simulink model "test_loopback_buf"  (Simulink 6.2)
settings: Solver=ode45  StartTime=0.0  StopTime=4000  RelTol=1e-3
undefined symbols (not defined in the file): Down, Up
libraries: xbsIndex_r3 x1383, xps_library x52, casper_library x37
(part 1 of 8)
settings Model: LastModifiedBy=dsp
settings DebuggingCC: SolverPrmCheckMsg=warning

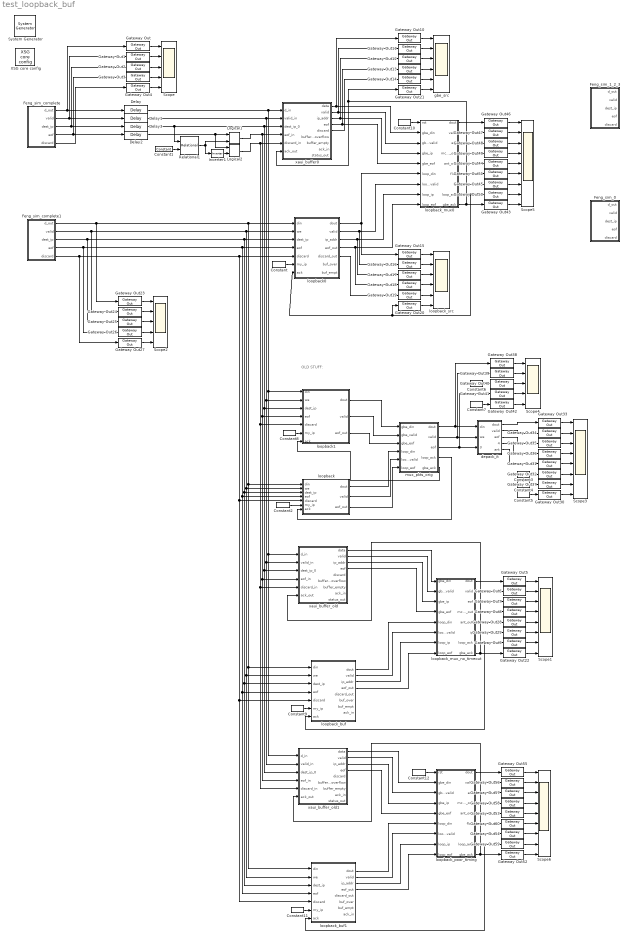
== system test_loopback_buf ==
  note: OLD STUFF:
  " System Generator" : xbsIndex_r3/ System Generator  Tag=genX  xilinxfamily=Virtex2P  part=xc2vp70  speed=-7  package=ff1704  synthesis_tool=XST  directory=./b_2x_8a_r308d/sysgen  testbench=off  simulink_period=1  sysclk_period=4.878  incr_netlist=off  trim_vbits=Everywhere in SubSystem  dbl_ovrd=According to Block Masks  core_generation=According to Block Masks  run_coregen=off  deprecated_control=off  eval_field=0
      settings: AttributesFormatString=System\nGenerator
  Constant{,1..12} (13 alike) : xbsIndex_r3/Constant  const=0  equ=P=C  arith_type=Unsigned  n_bits=1  bin_pt=0  opselect=C  inp2=PCIN>>17  opr=+  inp1=P  carry=CIN  iostate=0  explicit_period=on  period=1  dbl_ovrd=off
  Delay{,1..3} (4 alike) : xbsIndex_r3/Delay  latency=220  reg_retiming=off  explicit_period=off  period=1  en=off  accept_only_valid=off  init_zero=on  dbl_ovrd=off  show_param=off
      settings: xl_area=[0, 0, 0, 0, 0, 0, 0]
  Feng_sim_0 : Subsystem
  Feng_sim_1_2_3 : Subsystem
  Feng_sim_complete : Subsystem
  Feng_sim_complete1 : Subsystem
  Gateway Out{,1..60} (61 alike) : xbsIndex_r3/Gateway Out  output_type=Double  nbits=8  bin_pt=6  arith_type=Boolean  quantization=Truncate  overflow=Wrap  hdl_port=on  timing_constraint=None  locs_specified=off  LOCs={}  needs_fixed_name=off  show_param=off
      settings: xl_area=[0, 0, 0, 0, 0, 0, 0]
  Inverter1 : xbsIndex_r3/Inverter  latency=0  explicit_period=off  period=1  en=off  dbl_ovrd=off  show_param=off
      settings: xl_area=[0, 0, 0, 0, 0, 0, 0]
  Logical1 : xbsIndex_r3/Logical  logical_function=AND  inputs=2  precision=Full  arith_type=Unsigned  n_bits=8  bin_pt=2  align_bp=on  latency=0  explicit_period=off  period=1  en=off  dbl_ovrd=off  show_param=off
      settings: xl_area=[0, 0, 0, 0, 0, 0, 0]
  Logical2 : xbsIndex_r3/Logical  logical_function=AND  inputs=2  precision=Full  arith_type=Unsigned  n_bits=8  bin_pt=2  align_bp=on  latency=0  explicit_period=off  period=1  en=off  dbl_ovrd=off  show_param=off
      settings: xl_area=[0, 0, 0, 0, 0, 0, 0]
  Relational1 : xbsIndex_r3/Relational  mode=a!=b  latency=0  explicit_period=off  period=1  en=off  dbl_ovrd=off  show_param=off
      settings: xl_area=[0, 0, 0, 0, 0, 0, 0]
  Scope : Scope  NumInputPorts=5
      settings: TimeRange=10000  YMin=0~0~0~0~-1  YMax=5000~1~3~1~1
  Scope1 : Scope  NumInputPorts=8
      settings: YMin=1100~0~0~-1~0.95~-5~-5~-5  YMax=1200~1~1~1~1.05~5~5~5  SaveName=ScopeData19
  Scope2 : Scope  NumInputPorts=5
      settings: TimeRange=10000  YMin=0~0~0~0~-1  YMax=5000~1~3~1~1  SaveName=ScopeData12
  Scope3 : Scope  NumInputPorts=8
      settings: YMin=1100~0~0~-1~0.95~-5~-5~-5  YMax=1200~1~1~1~1.05~5~5~5  SaveName=ScopeData10
  Scope4 : Scope  NumInputPorts=5
      settings: TimeRange=10000  YMin=0~0~0~0~-1  YMax=5000~1~3~1~1  SaveName=ScopeData16
  Scope5 : Scope  NumInputPorts=9
      settings: YMin=1100~0~0~-1~0.95~-5~-5~-5~-5  YMax=1200~1~1~1~1.05~5~5~5~5  SaveName=ScopeData17
  Scope6 : Scope  NumInputPorts=9
      settings: YMin=1100~0~0~-1~0.95~-5~-5~-5~-5  YMax=1200~1~1~1~1.05~5~5~5~5  SaveName=ScopeData20
  XSG core config : xps_library/XSG core config  Tag=xps:xsg  hw_sys=BEE2_usr  ibob_linux=off  clk_src=sys_clk2x  gpio_clk_io_group=iBOB:sma  gpio_clk_bit_index=0  clk_rate=205  sample_period=1  synthesis_tool=XST  mpc_type=powerpc405
  depack_it : Subsystem  mask{payload_len=50}
      mask prompts: payload_len "Payload Length"
      mask init:
      | payload_bits = ceil(log2(payload_len));
      | packet_len = payload_len + 1;
      | packet_bits = ceil(log2(packet_len));
  gbe_src : Scope  NumInputPorts=6
      settings: YMin=95.95~0.95~1.9~-1~-1~-1  YMax=106.05~1.05~2.1~1~1~1  SaveName=ScopeData4
  loopback : Subsystem  mask{depth_bits=8}
      mask prompts: depth_bits "Buffer Size (2^?):"
      mask help: A loopback is a buffer for holding packets which are to be transmitted to one's self. Most switches drop any packets which have a destination IP address equal to the address of the transmitter. Thus, a seperate buffer is needed to collect these packets for readback.
  loopback0 : Subsystem  mask{depth_bits=10}
      mask prompts: depth_bits "Buffer Size (2^?):"
      mask help: A loopback is a buffer for holding packets which are to be transmitted to one's self. Most switches drop any packets which have a destination IP address equal to the address of the transmitter. Thus, a seperate buffer is needed to collect these packets for readback.
  loopback1 : Subsystem  mask{depth_bits=8}
      mask prompts: depth_bits "Buffer Size (2^?):"
      mask help: A loopback is a buffer for holding packets which are to be transmitted to one's self. Most switches drop any packets which have a destination IP address equal to the address of the transmitter. Thus, a seperate buffer is needed to collect these packets for readback.
  loopback_buf : Subsystem  mask{depth_bits=10}
      mask prompts: depth_bits "Buffer Size (2^?):"
      mask help: A loopback is a buffer for holding packets which are to be transmitted to one's self. Most switches drop any packets which have a destination IP address equal to the address of the transmitter. Thus, a seperate buffer is needed to collect these packets for readback.
  loopback_buf1 : Subsystem  mask{depth_bits=10}
      mask prompts: depth_bits "Buffer Size (2^?):"
      mask help: A loopback is a buffer for holding packets which are to be transmitted to one's self. Most switches drop any packets which have a destination IP address equal to the address of the transmitter. Thus, a seperate buffer is needed to collect these packets for readback.
  loopback_mux0 : Subsystem  mask{timeout_bits=27, payload_len=32}
      mask prompts: timeout_bits "Timeout (clock cycles, 2^?)"; payload_len "Expected payload length (in 64bit words)"
      mask init:
      | fmtstr = sprintf('Payload Len: %i', payload_len);
      | set_param(gcb, 'AttributesFormatString', fmtstr);
      settings: AttributesFormatString=Payload Len: 32
  loopback_mux_no_timeout : Subsystem  mask{loopback_timeout=20}
      mask prompts: loopback_timeout "loopback timeout (2^? clocks)"
  loopback_poor_timing : Subsystem  mask{timeout_bits=27, payload_len=50}
      mask prompts: timeout_bits "Timeout (clock cycles, 2^?)"; payload_len "Expected payload length (in 64bit words)"
      mask init:
      | fmtstr = sprintf('Payload Len: %i', payload_len);
      | set_param(gcb, 'AttributesFormatString', fmtstr);
      settings: AttributesFormatString=Payload Len: 50
  loopback_src : Scope  NumInputPorts=6
      settings: YMin=1500~0~1.59383e+008~0~-1~-5  YMax=3000~1~1.76161e+008~1~1~5  SaveName=ScopeData5
  mux_pkts_orig : Subsystem
  xaui_buffer0 : Subsystem  mask(mux_packets){depth_data_bits=10, depth_hdr_bits=5}
      mask prompts: depth_data_bits "Depth contents (2^?)"; depth_hdr_bits "Maximum number of packets to buffer? (2^?)"
      mask help: This block allows you to buffer a 10GbE datastream.
      mask init:
      | fmtstr = sprintf('Max %d data words.\nMax %d pkts.', 2^depth_data_bits,2^depth_hdr_bits);
      | set_param(gcb, 'AttributesFormatString', fmtstr);
      settings: AttributesFormatString=|
      | Max 1024 data words.
      | Max 32 pkts.
  xaui_buffer_old : Subsystem  mask(mux_packets){depth_data_bits=10, depth_hdr_bits=8}
      mask prompts: depth_data_bits "Depth contents (2^?)"; depth_hdr_bits "Maximum number of packets to buffer? (2^?)"
      mask help: This block allows you to buffer a 10GbE datastream.
      mask init:
      | fmtstr = sprintf('Max %d data words.\nMax %d pkts.', 2^depth_data_bits,2^depth_hdr_bits);
      | set_param(gcb, 'AttributesFormatString', fmtstr);
      settings: AttributesFormatString=|
      | Max 1024 data words.
      | Max 256 pkts.
  xaui_buffer_old1 : Subsystem  mask(mux_packets){depth_data_bits=10, depth_hdr_bits=8}
      mask prompts: depth_data_bits "Depth contents (2^?)"; depth_hdr_bits "Maximum number of packets to buffer? (2^?)"
      mask help: This block allows you to buffer a 10GbE datastream.
      mask init:
      | fmtstr = sprintf('Max %d data words.\nMax %d pkts.', 2^depth_data_bits,2^depth_hdr_bits);
      | set_param(gcb, 'AttributesFormatString', fmtstr);
      settings: AttributesFormatString=|
      | Max 1024 data words.
      | Max 256 pkts.
  wires:
  Feng_sim_complete/1(d_out) -> Gateway Out/1, Delay/1
  Feng_sim_complete/2(valid) -> Gateway Out1/1, Delay1/1
  Feng_sim_complete/4(eof) -> Gateway Out3/1, Delay2/1
  Feng_sim_complete/3(dest_ip) -> Gateway Out2/1, Delay3/1
  Feng_sim_complete/5(discard) -> Gateway Out4/1
  Gateway Out/1 -> Scope/1
  Gateway Out1/1 -> Scope/2
  Gateway Out2/1 -> Scope/3
  Gateway Out3/1 -> Scope/4
  Gateway Out4/1 -> Scope/5
  Delay/1 -> loopback1/1(din), xaui_buffer_old/1(d_in), xaui_buffer_old1/1(d_in), xaui_buffer0/1(d_in)
  Delay1/1 -> loopback1/2(we), xaui_buffer_old/2(valid_in), xaui_buffer_old1/2(valid_in), xaui_buffer0/2(valid_in)
  Delay3/1 -> Relational1/1, loopback1/3(dest_ip), xaui_buffer_old/3(dest_ip_0), xaui_buffer_old1/3(dest_ip_0), xaui_buffer0/3(dest_ip_0)
  Inverter1/1 -> Logical2/2
  Relational1/1 -> Inverter1/1, Logical1/2
  Logical1/1 -> loopback1/4(eof), xaui_buffer_old/4(eof_in), xaui_buffer_old1/4(eof_in), xaui_buffer0/4(eof_in)
  Logical2/1 -> loopback1/5(discard), xaui_buffer_old/5(discard_in), xaui_buffer_old1/5(discard_in), xaui_buffer0/5(discard_in)
  Constant1/1 -> Relational1/2
  Delay2/1 -> Logical1/1, Logical2/1
  Gateway Out10/1 -> gbe_src/1
  Gateway Out11/1 -> gbe_src/2
  Gateway Out12/1 -> gbe_src/3
  Gateway Out13/1 -> gbe_src/4
  Gateway Out14/1 -> gbe_src/5
  Gateway Out21/1 -> gbe_src/6
  Constant/1 -> loopback0/6(my_ip)
  Feng_sim_complete1/1(d_out) -> Gateway Out23/1, loopback/1(din), loopback_buf/1(din), loopback_buf1/1(din), loopback0/1(din)
  Feng_sim_complete1/2(valid) -> Gateway Out24/1, loopback/2(we), loopback_buf/2(we), loopback_buf1/2(we), loopback0/2(we)
  Feng_sim_complete1/3(dest_ip) -> Gateway Out25/1, loopback/3(dest_ip), loopback_buf/3(dest_ip), loopback_buf1/3(dest_ip), loopback0/3(dest_ip)
  Feng_sim_complete1/4(eof) -> Gateway Out26/1, loopback/4(eof), loopback_buf/4(eof), loopback_buf1/4(eof), loopback0/4(eof)
  Feng_sim_complete1/5(discard) -> Gateway Out27/1, loopback/5(discard), loopback_buf/5(discard), loopback_buf1/5(discard), loopback0/5(discard)
  Gateway Out23/1 -> Scope2/1
  Gateway Out24/1 -> Scope2/2
  Gateway Out25/1 -> Scope2/3
  Gateway Out26/1 -> Scope2/4
  Gateway Out27/1 -> Scope2/5
  mux_pkts_orig/1(dout) -> depack_it/1(din), Gateway Out38/1
  mux_pkts_orig/2(valid) -> depack_it/2(we), Gateway Out39/1
  mux_pkts_orig/3(eof) -> depack_it/3(eof_in), Gateway Out41/1
  loopback/1(dout) -> mux_pkts_orig/4(loop_din)
  loopback/2(valid) -> mux_pkts_orig/5(loop_valid)
  loopback/3(eof_out) -> mux_pkts_orig/6(loop_eof)
  mux_pkts_orig/4(loop_ack) -> loopback/7(ack)
  loopback1/1(dout) -> mux_pkts_orig/1(gbe_din)
  loopback1/2(valid) -> mux_pkts_orig/2(gbe_valid)
  loopback1/3(eof_out) -> mux_pkts_orig/3(gbe_eof)
  Constant2/1 -> loopback/6(my_ip)
  Gateway Out33/1 -> Scope3/1
  Gateway Out34/1 -> Scope3/2
  Gateway Out35/1 -> Scope3/3
  Gateway Out36/1 -> Scope3/4
  Gateway Out31/1 -> Scope3/5
  Gateway Out32/1 -> Scope3/6
  Gateway Out37/1 -> Scope3/7
  Gateway Out30/1 -> Scope3/8
  depack_it/1(dout) -> Gateway Out33/1
  depack_it/2(valid) -> Gateway Out34/1
  depack_it/3(eof) -> Gateway Out35/1
  depack_it/4(mcnt) -> Gateway Out36/1
  depack_it/5(ant) -> Gateway Out31/1
  Constant3/1 -> Gateway Out32/1
  Constant4/1 -> Gateway Out37/1
  Constant5/1 -> Gateway Out30/1
  Gateway Out38/1 -> Scope4/1
  Gateway Out39/1 -> Scope4/2
  Gateway Out40/1 -> Scope4/3
  Gateway Out41/1 -> Scope4/4
  Gateway Out42/1 -> Scope4/5
  Constant6/1 -> Gateway Out40/1
  Constant7/1 -> Gateway Out42/1
  Constant8/1 -> loopback1/6(my_ip)
  mux_pkts_orig/5(gbe_ack) -> loopback1/7(ack)
  Constant9/1 -> loopback_buf/6(my_ip)
  Gateway Out46/1 -> Scope5/1
  Gateway Out47/1 -> Scope5/2
  Gateway Out48/1 -> Scope5/3
  Gateway Out49/1 -> Scope5/4
  Gateway Out44/1 -> Scope5/5
  xaui_buffer0/1(data) -> Gateway Out10/1, loopback_mux0/2(gbe_din)
  xaui_buffer0/2(valid) -> Gateway Out11/1, loopback_mux0/3(gbe_valid)
  xaui_buffer0/3(ip_addr) -> Gateway Out12/1, loopback_mux0/4(gbe_ip)
  xaui_buffer0/4(eof) -> Gateway Out13/1, loopback_mux0/5(gbe_eof)
  loopback0/1(dout) -> Gateway Out15/1, loopback_mux0/6(loop_din)
  loopback0/2(valid) -> Gateway Out16/1, loopback_mux0/7(loop_valid)
  loopback0/3(ip_addr) -> Gateway Out17/1, loopback_mux0/8(loop_ip)
  loopback0/4(eof_out) -> Gateway Out18/1, loopback_mux0/9(loop_eof)
  Constant10/1 -> loopback_mux0/1(rst)
  Gateway Out5/1 -> Scope1/1
  Gateway Out6/1 -> Scope1/2
  Gateway Out7/1 -> Scope1/3
  xaui_buffer_old/1(data) -> loopback_mux_no_timeout/1(gbe_din)
  xaui_buffer_old/2(valid) -> loopback_mux_no_timeout/2(gbe_valid)
  xaui_buffer_old/4(eof) -> loopback_mux_no_timeout/4(gbe_eof)
  xaui_buffer_old/3(ip_addr) -> loopback_mux_no_timeout/3(gbe_ip)
  loopback_buf/2(valid) -> loopback_mux_no_timeout/6(loop_valid)
  loopback_buf/3(ip_addr) -> loopback_mux_no_timeout/7(loop_ip)
  loopback_buf/4(eof_out) -> loopback_mux_no_timeout/8(loop_eof)
  loopback_mux_no_timeout/7(loop_ack) -> Gateway Out9/1, loopback_buf/7(ack)
  loopback_mux_no_timeout/8(gbe_ack) -> Gateway Out22/1, xaui_buffer_old/6(ack_out)
  loopback_mux_no_timeout/1(dout) -> Gateway Out5/1
  loopback_mux_no_timeout/2(valid) -> Gateway Out6/1
  loopback_mux_no_timeout/3(eof) -> Gateway Out7/1
  Gateway Out8/1 -> Scope1/4
  Gateway Out28/1 -> Scope1/5
  Gateway Out29/1 -> Scope1/6
  Gateway Out9/1 -> Scope1/7
  Gateway Out22/1 -> Scope1/8
  loopback_mux_no_timeout/4(mcnt_out) -> Gateway Out8/1
  loopback_mux_no_timeout/5(ant_out) -> Gateway Out28/1
  loopback_mux_no_timeout/6(ip) -> Gateway Out29/1
  xaui_buffer0/5(discard) -> Gateway Out14/1
  loopback_buf/1(dout) -> loopback_mux_no_timeout/5(loop_din)
  Gateway Out15/1 -> loopback_src/1
  Gateway Out16/1 -> loopback_src/2
  Gateway Out17/1 -> loopback_src/3
  Gateway Out18/1 -> loopback_src/4
  Gateway Out19/1 -> loopback_src/5
  Gateway Out20/1 -> loopback_src/6
  Gateway Out51/1 -> Scope5/6
  Gateway Out45/1 -> Scope5/7
  Gateway Out50/1 -> Scope5/8
  Gateway Out43/1 -> Scope5/9
  loopback_mux0/1(dout) -> Gateway Out46/1
  loopback_mux0/2(valid) -> Gateway Out47/1
  loopback_mux0/3(eof) -> Gateway Out48/1
  loopback_mux0/4(mcnt_out) -> Gateway Out49/1
  loopback_mux0/5(ant_out) -> Gateway Out44/1
  loopback_mux0/6(flag) -> Gateway Out51/1
  loopback_mux0/7(ip) -> Gateway Out45/1
  loopback_mux0/8(loop_ack) -> Gateway Out50/1, Gateway Out20/1, loopback0/7(ack)
  loopback_mux0/9(gbe_ack) -> Gateway Out43/1, Gateway Out21/1, xaui_buffer0/6(ack_out)
  Constant11/1 -> loopback_buf1/6(my_ip)
  xaui_buffer_old1/1(data) -> loopback_poor_timing/2(gbe_din)
  xaui_buffer_old1/2(valid) -> loopback_poor_timing/3(gbe_valid)
  xaui_buffer_old1/4(eof) -> loopback_poor_timing/5(gbe_eof)
  xaui_buffer_old1/3(ip_addr) -> loopback_poor_timing/4(gbe_ip)
  loopback_poor_timing/8(loop_ack) -> loopback_buf1/7(ack), Gateway Out59/1
  loopback_poor_timing/9(gbe_ack) -> xaui_buffer_old1/6(ack_out), Gateway Out52/1
  loopback_buf1/2(valid) -> loopback_poor_timing/7(loop_valid)
  loopback_buf1/3(ip_addr) -> loopback_poor_timing/8(loop_ip)
  loopback_buf1/4(eof_out) -> loopback_poor_timing/9(loop_eof)
  loopback_buf1/1(dout) -> loopback_poor_timing/6(loop_din)
  Gateway Out55/1 -> Scope6/1
  Gateway Out56/1 -> Scope6/2
  Gateway Out57/1 -> Scope6/3
  Gateway Out58/1 -> Scope6/4
  Gateway Out53/1 -> Scope6/5
  Gateway Out60/1 -> Scope6/6
  Gateway Out54/1 -> Scope6/7
  Gateway Out59/1 -> Scope6/8
  Gateway Out52/1 -> Scope6/9
  Constant12/1 -> loopback_poor_timing/1(rst)
  loopback_poor_timing/1(dout) -> Gateway Out55/1
  loopback_poor_timing/2(valid) -> Gateway Out56/1
  loopback_poor_timing/3(eof) -> Gateway Out57/1
  loopback_poor_timing/4(mcnt_out) -> Gateway Out58/1
  loopback_poor_timing/5(ant_out) -> Gateway Out53/1
  loopback_poor_timing/6(flag) -> Gateway Out60/1
  loopback_poor_timing/7(ip) -> Gateway Out54/1
  loopback0/5(discard_out) -> Gateway Out19/1

== system test_loopback_buf/Feng_sim_0 ==
  Concat1 : xbsIndex_r3/Concat  num_inputs=3  explicit_period=off  period=1  dbl_ovrd=off
  Constant : xbsIndex_r3/Constant  const=0  equ=P=C  arith_type=Boolean  n_bits=1  bin_pt=0  opselect=C  inp2=PCIN>>17  opr=+  inp1=P  carry=CIN  iostate=0  explicit_period=on  period=1  dbl_ovrd=off
  Constant1 : xbsIndex_r3/Constant  const=1  equ=P=C  arith_type=Boolean  n_bits=1  bin_pt=0  opselect=C  inp2=PCIN>>17  opr=+  inp1=P  carry=CIN  iostate=0  explicit_period=off  period=1  dbl_ovrd=off
  Constant2 : Constant
  Constant3 : xbsIndex_r3/Constant  const=0  equ=P=C  arith_type=Boolean  n_bits=1  bin_pt=0  opselect=C  inp2=PCIN>>17  opr=+  inp1=P  carry=CIN  iostate=0  explicit_period=off  period=1  dbl_ovrd=off
  Constant4 : xbsIndex_r3/Constant  const=0  equ=P=C  arith_type=Unsigned  n_bits=32  bin_pt=0  opselect=C  inp2=PCIN>>17  opr=+  inp1=P  carry=CIN  iostate=0  explicit_period=on  period=1  dbl_ovrd=off
  Constant5 : xbsIndex_r3/Constant  const=0  equ=P=C  arith_type=Unsigned  n_bits=16-2  bin_pt=0  opselect=C  inp2=PCIN>>17  opr=+  inp1=P  carry=CIN  iostate=0  explicit_period=on  period=1  dbl_ovrd=off
  Constant6 : xbsIndex_r3/Constant  const=0  equ=P=C  arith_type=Unsigned  n_bits=32  bin_pt=0  opselect=C  inp2=PCIN>>17  opr=+  inp1=P  carry=CIN  iostate=0  explicit_period=on  period=1  dbl_ovrd=off
  Convert1 : xbsIndex_r3/Convert  arith_type=Boolean  n_bits=8  bin_pt=6  quantization=Truncate  overflow=Wrap  latency=0  explicit_period=on  period=1  dbl_ovrd=off  show_param=off  inserted_by_tool=off  pipeline=off
      settings: xl_area=[0, 0, 0, 0, 0, 0, 0]
  Convert2 : xbsIndex_r3/Convert  arith_type=Boolean  n_bits=8  bin_pt=6  quantization=Truncate  overflow=Wrap  latency=0  explicit_period=on  period=1  dbl_ovrd=off  show_param=off  inserted_by_tool=off  pipeline=off
      settings: xl_area=[0, 0, 0, 0, 0, 0, 0]
  Convert3 : xbsIndex_r3/Convert  arith_type=Boolean  n_bits=8  bin_pt=6  quantization=Truncate  overflow=Wrap  latency=0  explicit_period=on  period=1  dbl_ovrd=off  show_param=off  inserted_by_tool=off  pipeline=off
      settings: xl_area=[0, 0, 0, 0, 0, 0, 0]
  Counter1 : xbsIndex_r3/Counter  cnt_type=Free Running  n_bits=64  bin_pt=0  arith_type=Unsigned  start_count=0  cnt_to=Inf  cnt_by_val=1  operation=Up  explicit_period=off  period=1  load_pin=off  rst=on  en=on  dbl_ovrd=off  show_param=off  use_rpm=off  gen_core=off
      settings: xl_area=[0, 0, 0, 0, 0, 0, 0]
  Counter2 : xbsIndex_r3/Counter  cnt_type=Free Running  n_bits=32  bin_pt=0  arith_type=Unsigned  start_count=1  cnt_to=Inf  cnt_by_val=1  operation=Up  explicit_period=on  period=1  load_pin=off  rst=on  en=off  dbl_ovrd=off  show_param=off  use_rpm=on  gen_core=off
      settings: xl_area=[0, 0, 0, 0, 0, 0, 0]
  Counter3 : xbsIndex_r3/Counter  cnt_type=Free Running  n_bits=32  bin_pt=0  arith_type=Unsigned  start_count=0  cnt_to=1023  cnt_by_val=1  operation=Up  explicit_period=on  period=1  load_pin=off  rst=on  en=on  dbl_ovrd=off  show_param=off  use_rpm=on  gen_core=off
      settings: xl_area=[0, 0, 0, 0, 0, 0, 0]
  Delay{1..2,4..5,8} (5 alike) : xbsIndex_r3/Delay  latency=1  reg_retiming=on  explicit_period=off  period=1  en=off  accept_only_valid=off  init_zero=on  dbl_ovrd=off  show_param=off
      settings: xl_area=[0, 0, 0, 0, 0, 0, 0]
  Gateway Out{,1..4} (5 alike) : xbsIndex_r3/Gateway Out  output_type=Double  nbits=8  bin_pt=6  arith_type=Boolean  quantization=Truncate  overflow=Wrap  hdl_port=on  timing_constraint=None  locs_specified=off  LOCs={}  needs_fixed_name=off  show_param=off
      settings: xl_area=[0, 0, 0, 0, 0, 0, 0]
  Inverter : xbsIndex_r3/Inverter  latency=0  explicit_period=off  period=1  en=off  dbl_ovrd=off  show_param=off
      settings: xl_area=[0, 0, 0, 0, 0, 0, 0]
  Inverter1 : xbsIndex_r3/Inverter  latency=0  explicit_period=off  period=1  en=off  dbl_ovrd=off  show_param=off
      settings: xl_area=[0, 0, 0, 0, 0, 0, 0]
  Inverter2 : xbsIndex_r3/Inverter  latency=0  explicit_period=off  period=1  en=off  dbl_ovrd=off  show_param=off
      settings: xl_area=[0, 0, 0, 0, 0, 0, 0]
  Logical : xbsIndex_r3/Logical  logical_function=AND  inputs=2  precision=Full  arith_type=Unsigned  n_bits=8  bin_pt=2  align_bp=on  latency=0  explicit_period=off  period=1  en=off  dbl_ovrd=off  show_param=off
      settings: xl_area=[0, 0, 0, 0, 0, 0, 0]
  Mux{,1..3} (4 alike) : xbsIndex_r3/Mux  inputs=2  precision=Full  arith_type="Signed  (2's comp)"  n_bits=8  bin_pt=2  quantization=Truncate  overflow=Wrap  latency=1  explicit_period=off  period=1  en=off  dbl_ovrd=off  show_param=off  mux_type=off  use_rpm=off  gen_core=off
      settings: xl_area=[0, 0, 0, 0, 0, 0, 0]
  Relational : xbsIndex_r3/Relational  mode=a>=b  latency=0  explicit_period=on  period=1  en=off  dbl_ovrd=off  show_param=off
      settings: xl_area=[0, 0, 0, 0, 0, 0, 0]
  Relational1 : xbsIndex_r3/Relational  mode=a=b  latency=0  explicit_period=off  period=1  en=off  dbl_ovrd=off  show_param=off
      settings: xl_area=[0, 0, 0, 0, 0, 0, 0]
  Relational5 : xbsIndex_r3/Relational  mode=a<=b  latency=0  explicit_period=off  period=1  en=off  dbl_ovrd=off  show_param=off
      settings: xl_area=[0, 0, 0, 0, 0, 0, 0]
  Scope : Scope  NumInputPorts=5
      settings: TimeRange=4000  YMin=130000~0~0~0~0  YMax=200000~1~1~1~1  SaveName=ScopeData11
  Slice1 : xbsIndex_r3/Slice  mode=Lower Bit Location + Width  nbits=1  bit1=1  base1=MSB of Input  bit0=0  base0=LSB of Input  boolean_output=off  explicit_period=off  period=1  dbl_ovrd=off
  Slice2 : xbsIndex_r3/Slice  mode=Lower Bit Location + Width  nbits=2  bit1=1  base1=MSB of Input  bit0=0  base0=LSB of Input  boolean_output=off  explicit_period=off  period=1  dbl_ovrd=off
  Slice3 : xbsIndex_r3/Slice  mode=Lower Bit Location + Width  nbits=48  bit1=1  base1=MSB of Input  bit0=2  base0=LSB of Input  boolean_output=off  explicit_period=off  period=1  dbl_ovrd=off
  mcnt_cnt : xbsIndex_r3/Counter  cnt_type=Free Running  n_bits=64  bin_pt=0  arith_type=Unsigned  start_count=0  cnt_to=Inf  cnt_by_val=1  operation=Up  explicit_period=off  period=1  load_pin=off  rst=off  en=on  dbl_ovrd=off  show_param=off  use_rpm=off  gen_core=off
      settings: xl_area=[0, 0, 0, 0, 0, 0, 0]
  negedge : casper_library/Misc/negedge  Tag=Rising Edge Detector
  payload_len : xps_library/software register  Tag=xps:sw_reg  io_dir=From Processor  arith_type=Unsigned  bitwidth=32  bin_pt=0  sample_period=1  gw_name=test_loopback_buf_Feng_sim_0_payload_len_user_data_out
  period : xps_library/software register  Tag=xps:sw_reg  io_dir=From Processor  arith_type=Unsigned  bitwidth=32  bin_pt=0  sample_period=1  gw_name=test_loopback_buf_Feng_sim_0_period_user_data_out
  posedge : casper_library/Misc/pulse_ext/posedge  Tag=Rising Edge Detector
  run : xps_library/software register  Tag=xps:sw_reg  io_dir=From Processor  arith_type=Unsigned  bitwidth=32  bin_pt=0  sample_period=1  gw_name=test_loopback_buf_Feng_sim_0_run_user_data_out
  sim_freq : Constant  Value=100
  sim_length : Constant  Value=50
  d_out : Outport
  valid : Outport  Port=2
  dest_ip : Outport  Port=3
  eof : Outport  Port=4
  discard : Outport  Port=5
  wires:
  Delay1/1 -> Delay8/1
  Slice2/1 -> Concat1/3
  Slice3/1 -> Concat1/1
  Logical/1 -> Gateway Out3/1, Delay2/1
  Gateway Out4/1 -> Scope/5
  Gateway Out3/1 -> Scope/4
  Gateway Out2/1 -> Scope/3
  Gateway Out1/1 -> Scope/2
  Gateway Out/1 -> Scope/1
  Delay5/1 -> Gateway Out4/1, Mux3/1
  Concat1/1 -> Gateway Out/1, Mux3/2
  Constant5/1 -> Concat1/2
  mcnt_cnt/1 -> Slice3/1
  Inverter2/1 -> Logical/1, Delay5/1
  Relational1/1 -> Inverter2/1
  Constant4/1 -> Relational1/1
  Constant6/1 -> Slice2/1, Delay1/1
  Convert2/1 -> Delay4/1
  Inverter1/1 -> Convert2/1
  Constant1/1 -> Mux2/3
  Constant3/1 -> Mux2/2
  Convert3/1 -> Inverter/1
  Delay2/1 -> Counter1/2
  Inverter/1 -> Counter1/1
  Mux2/1 -> Mux/3
  Delay4/1 -> discard/1
  Slice1/1 -> Convert3/1, Inverter1/1, Mux1/1, Mux/1
  Constant2/1 -> run/1
  run/1 -> Slice1/1
  Delay8/1 -> dest_ip/1
  Mux3/1 -> d_out/1
  Convert1/1 -> Mux1/3
  Mux1/1 -> eof/1
  Constant/1 -> Mux1/2, Mux/2
  Mux/1 -> Gateway Out2/1, valid/1
  payload_len/1 -> Relational5/2
  sim_length/1 -> payload_len/1
  posedge/1 -> Gateway Out1/1, mcnt_cnt/1, Counter3/1
  Counter3/1 -> Relational1/2, Relational5/1
  Relational5/1 -> Counter3/2, negedge/1, Mux2/1, Logical/2
  sim_freq/1 -> period/1
  period/1 -> Relational/2
  negedge/1 -> Convert1/1
  Counter1/1 -> Mux3/3
  Relational/1 -> Counter2/1, posedge/1
  Counter2/1 -> Relational/1

== system test_loopback_buf/Feng_sim_1_2_3 ==
  AddSub : xbsIndex_r3/AddSub  mode=Addition  precision=Full  arith_type=Unsigned  n_bits=8  bin_pt=2  quantization=Truncate  overflow=Wrap  latency=0  explicit_period=off  period=1  use_carryin=off  use_carryout=off  en=off  dbl_ovrd=off  show_param=off  use_core=on  pipeline=off  use_rpm=on  gen_core=off
      settings: xl_area=[0, 0, 0, 0, 0, 0, 0]
  Concat1 : xbsIndex_r3/Concat  num_inputs=3  explicit_period=off  period=1  dbl_ovrd=off
  Constant : xbsIndex_r3/Constant  const=0  equ=P=C  arith_type=Boolean  n_bits=1  bin_pt=0  opselect=C  inp2=PCIN>>17  opr=+  inp1=P  carry=CIN  iostate=0  explicit_period=on  period=1  dbl_ovrd=off
  Constant1 : xbsIndex_r3/Constant  const=1  equ=P=C  arith_type=Boolean  n_bits=1  bin_pt=0  opselect=C  inp2=PCIN>>17  opr=+  inp1=P  carry=CIN  iostate=0  explicit_period=off  period=1  dbl_ovrd=off
  Constant2 : Constant
  Constant3 : xbsIndex_r3/Constant  const=0  equ=P=C  arith_type=Boolean  n_bits=1  bin_pt=0  opselect=C  inp2=PCIN>>17  opr=+  inp1=P  carry=CIN  iostate=0  explicit_period=off  period=1  dbl_ovrd=off
  Constant4 : xbsIndex_r3/Constant  const=0  equ=P=C  arith_type=Unsigned  n_bits=32  bin_pt=0  opselect=C  inp2=PCIN>>17  opr=+  inp1=P  carry=CIN  iostate=0  explicit_period=on  period=1  dbl_ovrd=off
  Constant5 : xbsIndex_r3/Constant  const=0  equ=P=C  arith_type=Unsigned  n_bits=16-2  bin_pt=0  opselect=C  inp2=PCIN>>17  opr=+  inp1=P  carry=CIN  iostate=0  explicit_period=on  period=1  dbl_ovrd=off
  Convert1 : xbsIndex_r3/Convert  arith_type=Boolean  n_bits=8  bin_pt=6  quantization=Truncate  overflow=Wrap  latency=0  explicit_period=on  period=1  dbl_ovrd=off  show_param=off  inserted_by_tool=off  pipeline=off
      settings: xl_area=[0, 0, 0, 0, 0, 0, 0]
  Convert2 : xbsIndex_r3/Convert  arith_type=Boolean  n_bits=8  bin_pt=6  quantization=Truncate  overflow=Wrap  latency=0  explicit_period=on  period=1  dbl_ovrd=off  show_param=off  inserted_by_tool=off  pipeline=off
      settings: xl_area=[0, 0, 0, 0, 0, 0, 0]
  Convert3 : xbsIndex_r3/Convert  arith_type=Boolean  n_bits=8  bin_pt=6  quantization=Truncate  overflow=Wrap  latency=0  explicit_period=on  period=1  dbl_ovrd=off  show_param=off  inserted_by_tool=off  pipeline=off
      settings: xl_area=[0, 0, 0, 0, 0, 0, 0]
  Counter1 : xbsIndex_r3/Counter  cnt_type=Free Running  n_bits=64  bin_pt=0  arith_type=Unsigned  start_count=0  cnt_to=Inf  cnt_by_val=1  operation=Up  explicit_period=off  period=1  load_pin=off  rst=on  en=on  dbl_ovrd=off  show_param=off  use_rpm=off  gen_core=off
      settings: xl_area=[0, 0, 0, 0, 0, 0, 0]
  Counter2 : xbsIndex_r3/Counter  cnt_type=Free Running  n_bits=32  bin_pt=0  arith_type=Unsigned  start_count=1  cnt_to=Inf  cnt_by_val=1  operation=Up  explicit_period=on  period=1  load_pin=off  rst=on  en=off  dbl_ovrd=off  show_param=off  use_rpm=on  gen_core=off
      settings: xl_area=[0, 0, 0, 0, 0, 0, 0]
  Counter3 : xbsIndex_r3/Counter  cnt_type=Free Running  n_bits=32  bin_pt=0  arith_type=Unsigned  start_count=0  cnt_to=1023  cnt_by_val=1  operation=Up  explicit_period=on  period=1  load_pin=off  rst=on  en=on  dbl_ovrd=off  show_param=off  use_rpm=on  gen_core=off
      settings: xl_area=[0, 0, 0, 0, 0, 0, 0]
  Counter4 : xbsIndex_r3/Counter  cnt_type=Count Limited  n_bits=2  bin_pt=0  arith_type=Unsigned  start_count=0  cnt_to=2  cnt_by_val=1  operation=Up  explicit_period=on  period=1  load_pin=off  rst=off  en=on  dbl_ovrd=off  show_param=off  use_rpm=on  gen_core=off
      settings: xl_area=[0, 0, 0, 0, 0, 0, 0]
  Delay{1..2,4..5,8} (5 alike) : xbsIndex_r3/Delay  latency=1  reg_retiming=on  explicit_period=off  period=1  en=off  accept_only_valid=off  init_zero=on  dbl_ovrd=off  show_param=off
      settings: xl_area=[0, 0, 0, 0, 0, 0, 0]
  Gateway Out{,1..4} (5 alike) : xbsIndex_r3/Gateway Out  output_type=Double  nbits=8  bin_pt=6  arith_type=Boolean  quantization=Truncate  overflow=Wrap  hdl_port=on  timing_constraint=None  locs_specified=off  LOCs={}  needs_fixed_name=off  show_param=off
      settings: xl_area=[0, 0, 0, 0, 0, 0, 0]
  Inverter : xbsIndex_r3/Inverter  latency=0  explicit_period=off  period=1  en=off  dbl_ovrd=off  show_param=off
      settings: xl_area=[0, 0, 0, 0, 0, 0, 0]
  Inverter1 : xbsIndex_r3/Inverter  latency=0  explicit_period=off  period=1  en=off  dbl_ovrd=off  show_param=off
      settings: xl_area=[0, 0, 0, 0, 0, 0, 0]
  Inverter2 : xbsIndex_r3/Inverter  latency=0  explicit_period=off  period=1  en=off  dbl_ovrd=off  show_param=off
      settings: xl_area=[0, 0, 0, 0, 0, 0, 0]
  Logical : xbsIndex_r3/Logical  logical_function=AND  inputs=2  precision=Full  arith_type=Unsigned  n_bits=8  bin_pt=2  align_bp=on  latency=0  explicit_period=off  period=1  en=off  dbl_ovrd=off  show_param=off
      settings: xl_area=[0, 0, 0, 0, 0, 0, 0]
  Mux{,1..3} (4 alike) : xbsIndex_r3/Mux  inputs=2  precision=Full  arith_type="Signed  (2's comp)"  n_bits=8  bin_pt=2  quantization=Truncate  overflow=Wrap  latency=1  explicit_period=off  period=1  en=off  dbl_ovrd=off  show_param=off  mux_type=off  use_rpm=off  gen_core=off
      settings: xl_area=[0, 0, 0, 0, 0, 0, 0]
  Relational : xbsIndex_r3/Relational  mode=a>=b  latency=0  explicit_period=on  period=1  en=off  dbl_ovrd=off  show_param=off
      settings: xl_area=[0, 0, 0, 0, 0, 0, 0]
  Relational1 : xbsIndex_r3/Relational  mode=a=b  latency=0  explicit_period=off  period=1  en=off  dbl_ovrd=off  show_param=off
      settings: xl_area=[0, 0, 0, 0, 0, 0, 0]
  Relational5 : xbsIndex_r3/Relational  mode=a<=b  latency=0  explicit_period=off  period=1  en=off  dbl_ovrd=off  show_param=off
      settings: xl_area=[0, 0, 0, 0, 0, 0, 0]
  Scope : Scope  NumInputPorts=5
      settings: TimeRange=4000  YMin=130000~0~0~0~0  YMax=200000~1~1~1~1  SaveName=ScopeData11
  Slice : xbsIndex_r3/Slice  mode=Lower Bit Location + Width  nbits=31  bit1=0  base1=MSB of Input  bit0=0  base0=LSB of Input  boolean_output=off  explicit_period=off  period=1  dbl_ovrd=off
  Slice1 : xbsIndex_r3/Slice  mode=Lower Bit Location + Width  nbits=1  bit1=1  base1=MSB of Input  bit0=0  base0=LSB of Input  boolean_output=off  explicit_period=off  period=1  dbl_ovrd=off
  Slice2 : xbsIndex_r3/Slice  mode=Lower Bit Location + Width  nbits=2  bit1=1  base1=MSB of Input  bit0=0  base0=LSB of Input  boolean_output=off  explicit_period=off  period=1  dbl_ovrd=off
  Slice3 : xbsIndex_r3/Slice  mode=Lower Bit Location + Width  nbits=48  bit1=1  base1=MSB of Input  bit0=3  base0=LSB of Input  boolean_output=off  explicit_period=off  period=1  dbl_ovrd=off
  ip_addr : xps_library/software register  Tag=xps:sw_reg  io_dir=From Processor  arith_type=Unsigned  bitwidth=32  bin_pt=0  sample_period=1  gw_name=test_loopback_buf_Feng_sim_1_2_3_ip_addr_user_data_out
  mcnt_cnt : xbsIndex_r3/Counter  cnt_type=Free Running  n_bits=64  bin_pt=0  arith_type=Unsigned  start_count=0  cnt_to=Inf  cnt_by_val=1  operation=Up  explicit_period=off  period=1  load_pin=off  rst=off  en=on  dbl_ovrd=off  show_param=off  use_rpm=off  gen_core=off
      settings: xl_area=[0, 0, 0, 0, 0, 0, 0]
  negedge : casper_library/Misc/negedge  Tag=Rising Edge Detector
  payload_len : xps_library/software register  Tag=xps:sw_reg  io_dir=From Processor  arith_type=Unsigned  bitwidth=32  bin_pt=0  sample_period=1  gw_name=test_loopback_buf_Feng_sim_1_2_3_payload_len_user_data_out
  period : xps_library/software register  Tag=xps:sw_reg  io_dir=From Processor  arith_type=Unsigned  bitwidth=32  bin_pt=0  sample_period=1  gw_name=test_loopback_buf_Feng_sim_1_2_3_period_user_data_out
  posedge : casper_library/Misc/pulse_ext/posedge  Tag=Rising Edge Detector
  run : xps_library/software register  Tag=xps:sw_reg  io_dir=From Processor  arith_type=Unsigned  bitwidth=32  bin_pt=0  sample_period=1  gw_name=test_loopback_buf_Feng_sim_1_2_3_run_user_data_out
  sim_IP : Constant
  sim_freq : Constant  Value=52
  sim_length : Constant  Value=50
  d_out : Outport
  valid : Outport  Port=2
  dest_ip : Outport  Port=3
  eof : Outport  Port=4
  discard : Outport  Port=5
  wires:
  Counter2/1 -> Relational/1
  Relational/1 -> posedge/1, Counter2/1
  Counter1/1 -> Mux3/3
  negedge/1 -> Convert1/1
  period/1 -> Relational/2
  sim_freq/1 -> period/1
  sim_IP/1 -> ip_addr/1
  Relational5/1 -> Logical/2, Mux2/1, negedge/1, Counter3/2
  Counter3/1 -> Relational5/1, Relational1/2
  posedge/1 -> Counter3/1, Counter4/1, mcnt_cnt/1, Gateway Out1/1
  sim_length/1 -> payload_len/1
  payload_len/1 -> Relational5/2
  Mux/1 -> valid/1, Gateway Out2/1
  Constant/1 -> Mux/2, Mux1/2
  Mux1/1 -> eof/1
  Convert1/1 -> Mux1/3
  Mux3/1 -> d_out/1
  Delay8/1 -> dest_ip/1
  run/1 -> Slice1/1
  Constant2/1 -> run/1
  Slice1/1 -> Mux/1, Mux1/1, Inverter1/1, Convert3/1
  Delay4/1 -> discard/1
  Mux2/1 -> Mux/3
  Inverter/1 -> Counter1/1
  Delay2/1 -> Counter1/2
  Convert3/1 -> Inverter/1
  Constant3/1 -> Mux2/2
  Constant1/1 -> Mux2/3
  Inverter1/1 -> Convert2/1
  Convert2/1 -> Delay4/1
  ip_addr/1 -> Slice/1
  Slice/1 -> AddSub/1
  AddSub/1 -> Delay1/1, Slice2/1
  Constant4/1 -> Relational1/1
  Relational1/1 -> Inverter2/1
  Inverter2/1 -> Delay5/1, Logical/1
  mcnt_cnt/1 -> Slice3/1
  Constant5/1 -> Concat1/2
  Concat1/1 -> Mux3/2, Gateway Out/1
  Delay5/1 -> Mux3/1, Gateway Out4/1
  Gateway Out/1 -> Scope/1
  Gateway Out1/1 -> Scope/2
  Gateway Out2/1 -> Scope/3
  Gateway Out3/1 -> Scope/4
  Gateway Out4/1 -> Scope/5
  Logical/1 -> Delay2/1, Gateway Out3/1
  Slice3/1 -> Concat1/1
  Slice2/1 -> Concat1/3
  Delay1/1 -> Delay8/1
  Counter4/1 -> AddSub/2

== system test_loopback_buf/Feng_sim_complete ==
  Concat : xbsIndex_r3/Concat  num_inputs=2  explicit_period=off  period=1  dbl_ovrd=off
  Concat1 : xbsIndex_r3/Concat  num_inputs=3  explicit_period=off  period=1  dbl_ovrd=off
  Constant : xbsIndex_r3/Constant  const=0  equ=P=C  arith_type=Boolean  n_bits=1  bin_pt=0  opselect=C  inp2=PCIN>>17  opr=+  inp1=P  carry=CIN  iostate=0  explicit_period=on  period=1  dbl_ovrd=off
  Constant1 : xbsIndex_r3/Constant  const=1  equ=P=C  arith_type=Boolean  n_bits=1  bin_pt=0  opselect=C  inp2=PCIN>>17  opr=+  inp1=P  carry=CIN  iostate=0  explicit_period=off  period=1  dbl_ovrd=off
  Constant2 : Constant
  Constant3 : xbsIndex_r3/Constant  const=0  equ=P=C  arith_type=Boolean  n_bits=1  bin_pt=0  opselect=C  inp2=PCIN>>17  opr=+  inp1=P  carry=CIN  iostate=0  explicit_period=off  period=1  dbl_ovrd=off
  Constant4 : xbsIndex_r3/Constant  const=0  equ=P=C  arith_type=Unsigned  n_bits=32  bin_pt=0  opselect=C  inp2=PCIN>>17  opr=+  inp1=P  carry=CIN  iostate=0  explicit_period=on  period=1  dbl_ovrd=off
  Constant5 : xbsIndex_r3/Constant  const=0  equ=P=C  arith_type=Unsigned  n_bits=16-2  bin_pt=0  opselect=C  inp2=PCIN>>17  opr=+  inp1=P  carry=CIN  iostate=0  explicit_period=on  period=1  dbl_ovrd=off
  Convert1 : xbsIndex_r3/Convert  arith_type=Boolean  n_bits=8  bin_pt=6  quantization=Truncate  overflow=Wrap  latency=0  explicit_period=on  period=1  dbl_ovrd=off  show_param=off  inserted_by_tool=off  pipeline=off
      settings: xl_area=[0, 0, 0, 0, 0, 0, 0]
  Convert2 : xbsIndex_r3/Convert  arith_type=Boolean  n_bits=8  bin_pt=6  quantization=Truncate  overflow=Wrap  latency=0  explicit_period=on  period=1  dbl_ovrd=off  show_param=off  inserted_by_tool=off  pipeline=off
      settings: xl_area=[0, 0, 0, 0, 0, 0, 0]
  Convert3 : xbsIndex_r3/Convert  arith_type=Boolean  n_bits=8  bin_pt=6  quantization=Truncate  overflow=Wrap  latency=0  explicit_period=on  period=1  dbl_ovrd=off  show_param=off  inserted_by_tool=off  pipeline=off
      settings: xl_area=[0, 0, 0, 0, 0, 0, 0]
  Counter1 : xbsIndex_r3/Counter  cnt_type=Free Running  n_bits=64  bin_pt=0  arith_type=Unsigned  start_count=0  cnt_to=Inf  cnt_by_val=1  operation=Up  explicit_period=off  period=1  load_pin=off  rst=on  en=on  dbl_ovrd=off  show_param=off  use_rpm=off  gen_core=off
      settings: xl_area=[0, 0, 0, 0, 0, 0, 0]
  Counter2 : xbsIndex_r3/Counter  cnt_type=Free Running  n_bits=32  bin_pt=0  arith_type=Unsigned  start_count=1  cnt_to=Inf  cnt_by_val=1  operation=Up  explicit_period=on  period=1  load_pin=off  rst=on  en=off  dbl_ovrd=off  show_param=off  use_rpm=on  gen_core=off
      settings: xl_area=[0, 0, 0, 0, 0, 0, 0]
  Counter3 : xbsIndex_r3/Counter  cnt_type=Free Running  n_bits=32  bin_pt=0  arith_type=Unsigned  start_count=0  cnt_to=1023  cnt_by_val=1  operation=Up  explicit_period=on  period=1  load_pin=off  rst=on  en=on  dbl_ovrd=off  show_param=off  use_rpm=on  gen_core=off
      settings: xl_area=[0, 0, 0, 0, 0, 0, 0]
  Counter4 : xbsIndex_r3/Counter  cnt_type=Free Running  n_bits=2  bin_pt=0  arith_type=Unsigned  start_count=0  cnt_to=1023  cnt_by_val=1  operation=Up  explicit_period=on  period=1  load_pin=off  rst=off  en=on  dbl_ovrd=off  show_param=off  use_rpm=on  gen_core=off
      settings: xl_area=[0, 0, 0, 0, 0, 0, 0]
  Delay{1..2,4..5,8} (5 alike) : xbsIndex_r3/Delay  latency=1  reg_retiming=on  explicit_period=off  period=1  en=off  accept_only_valid=off  init_zero=on  dbl_ovrd=off  show_param=off
      settings: xl_area=[0, 0, 0, 0, 0, 0, 0]
  Gateway Out{,1..4} (5 alike) : xbsIndex_r3/Gateway Out  output_type=Double  nbits=8  bin_pt=6  arith_type=Boolean  quantization=Truncate  overflow=Wrap  hdl_port=on  timing_constraint=None  locs_specified=off  LOCs={}  needs_fixed_name=off  show_param=off
      settings: xl_area=[0, 0, 0, 0, 0, 0, 0]
  Inverter : xbsIndex_r3/Inverter  latency=0  explicit_period=off  period=1  en=off  dbl_ovrd=off  show_param=off
      settings: xl_area=[0, 0, 0, 0, 0, 0, 0]
  Inverter1 : xbsIndex_r3/Inverter  latency=0  explicit_period=off  period=1  en=off  dbl_ovrd=off  show_param=off
      settings: xl_area=[0, 0, 0, 0, 0, 0, 0]
  Inverter2 : xbsIndex_r3/Inverter  latency=0  explicit_period=off  period=1  en=off  dbl_ovrd=off  show_param=off
      settings: xl_area=[0, 0, 0, 0, 0, 0, 0]
  Logical : xbsIndex_r3/Logical  logical_function=AND  inputs=2  precision=Full  arith_type=Unsigned  n_bits=8  bin_pt=2  align_bp=on  latency=0  explicit_period=off  period=1  en=off  dbl_ovrd=off  show_param=off
      settings: xl_area=[0, 0, 0, 0, 0, 0, 0]
  Mux{,1..3} (4 alike) : xbsIndex_r3/Mux  inputs=2  precision=Full  arith_type="Signed  (2's comp)"  n_bits=8  bin_pt=2  quantization=Truncate  overflow=Wrap  latency=1  explicit_period=off  period=1  en=off  dbl_ovrd=off  show_param=off  mux_type=off  use_rpm=off  gen_core=off
      settings: xl_area=[0, 0, 0, 0, 0, 0, 0]
  Relational : xbsIndex_r3/Relational  mode=a>=b  latency=0  explicit_period=on  period=1  en=off  dbl_ovrd=off  show_param=off
      settings: xl_area=[0, 0, 0, 0, 0, 0, 0]
  Relational1 : xbsIndex_r3/Relational  mode=a=b  latency=0  explicit_period=off  period=1  en=off  dbl_ovrd=off  show_param=off
      settings: xl_area=[0, 0, 0, 0, 0, 0, 0]
  Relational5 : xbsIndex_r3/Relational  mode=a<=b  latency=0  explicit_period=off  period=1  en=off  dbl_ovrd=off  show_param=off
      settings: xl_area=[0, 0, 0, 0, 0, 0, 0]
  Scope : Scope  NumInputPorts=5
      settings: TimeRange=4000  YMin=130000~0~0~0~0  YMax=200000~1~1~1~1  SaveName=ScopeData11
  Slice : xbsIndex_r3/Slice  mode=Upper Bit Location + Width  nbits=30  bit1=0  base1=MSB of Input  bit0=0  base0=LSB of Input  boolean_output=off  explicit_period=off  period=1  dbl_ovrd=off
  Slice1 : xbsIndex_r3/Slice  mode=Lower Bit Location + Width  nbits=1  bit1=1  base1=MSB of Input  bit0=0  base0=LSB of Input  boolean_output=off  explicit_period=off  period=1  dbl_ovrd=off
  Slice2 : xbsIndex_r3/Slice  mode=Lower Bit Location + Width  nbits=2  bit1=1  base1=MSB of Input  bit0=0  base0=LSB of Input  boolean_output=off  explicit_period=off  period=1  dbl_ovrd=off
  Slice3 : xbsIndex_r3/Slice  mode=Lower Bit Location + Width  nbits=48  bit1=1  base1=MSB of Input  bit0=3  base0=LSB of Input  boolean_output=off  explicit_period=off  period=1  dbl_ovrd=off
  ip_addr : xps_library/software register  Tag=xps:sw_reg  io_dir=From Processor  arith_type=Unsigned  bitwidth=32  bin_pt=0  sample_period=1  gw_name=test_loopback_buf_Feng_sim_complete_ip_addr_user_data_out
  mcnt_cnt : xbsIndex_r3/Counter  cnt_type=Free Running  n_bits=64  bin_pt=0  arith_type=Unsigned  start_count=0  cnt_to=Inf  cnt_by_val=1  operation=Up  explicit_period=off  period=1  load_pin=off  rst=off  en=on  dbl_ovrd=off  show_param=off  use_rpm=off  gen_core=off
      settings: xl_area=[0, 0, 0, 0, 0, 0, 0]
  negedge : casper_library/Misc/negedge  Tag=Rising Edge Detector
  payload_len : xps_library/software register  Tag=xps:sw_reg  io_dir=From Processor  arith_type=Unsigned  bitwidth=32  bin_pt=0  sample_period=1  gw_name=test_loopback_buf_Feng_sim_complete_payload_len_user_data_out
  period : xps_library/software register  Tag=xps:sw_reg  io_dir=From Processor  arith_type=Unsigned  bitwidth=32  bin_pt=0  sample_period=1  gw_name=test_loopback_buf_Feng_sim_complete_period_user_data_out
  posedge : casper_library/Misc/pulse_ext/posedge  Tag=Rising Edge Detector
  run : xps_library/software register  Tag=xps:sw_reg  io_dir=From Processor  arith_type=Unsigned  bitwidth=32  bin_pt=0  sample_period=1  gw_name=test_loopback_buf_Feng_sim_complete_run_user_data_out
  sim_IP : Constant  Value=0
  sim_freq : Constant  Value=52
  sim_length : Constant  Value=50
  d_out : Outport
  valid : Outport  Port=2
  dest_ip : Outport  Port=3
  eof : Outport  Port=4
  discard : Outport  Port=5
  wires:
  Counter2/1 -> Relational/1
  Relational/1 -> posedge/1, Counter2/1
  Counter1/1 -> Mux3/3
  negedge/1 -> Convert1/1
  period/1 -> Relational/2
  sim_freq/1 -> period/1
  sim_IP/1 -> ip_addr/1
  Relational5/1 -> Logical/2, Mux2/1, negedge/1, Counter3/2
  Counter3/1 -> Relational5/1, Relational1/2
  posedge/1 -> Counter3/1, Counter4/1, mcnt_cnt/1, Gateway Out1/1
  sim_length/1 -> payload_len/1
  payload_len/1 -> Relational5/2
  Mux/1 -> valid/1, Gateway Out2/1
  Constant/1 -> Mux/2, Mux1/2
  Mux1/1 -> eof/1
  Convert1/1 -> Mux1/3
  Mux3/1 -> d_out/1
  Delay8/1 -> dest_ip/1
  run/1 -> Slice1/1
  Constant2/1 -> run/1
  Slice1/1 -> Mux/1, Mux1/1, Inverter1/1, Convert3/1
  Delay4/1 -> discard/1
  Mux2/1 -> Mux/3
  Inverter/1 -> Counter1/1
  Delay2/1 -> Counter1/2
  Convert3/1 -> Inverter/1
  Constant3/1 -> Mux2/2
  Constant1/1 -> Mux2/3
  Inverter1/1 -> Convert2/1
  Convert2/1 -> Delay4/1
  ip_addr/1 -> Slice/1
  Counter4/1 -> Concat/2
  Slice/1 -> Concat/1
  Concat/1 -> Delay1/1, Slice2/1
  Constant4/1 -> Relational1/1
  Relational1/1 -> Inverter2/1
  Inverter2/1 -> Delay5/1, Logical/1
  mcnt_cnt/1 -> Slice3/1
  Constant5/1 -> Concat1/2
  Concat1/1 -> Mux3/2, Gateway Out/1
  Delay5/1 -> Mux3/1, Gateway Out4/1
  Gateway Out/1 -> Scope/1
  Gateway Out1/1 -> Scope/2
  Gateway Out2/1 -> Scope/3
  Gateway Out3/1 -> Scope/4
  Gateway Out4/1 -> Scope/5
  Logical/1 -> Delay2/1, Gateway Out3/1
  Slice3/1 -> Concat1/1
  Slice2/1 -> Concat1/3
  Delay1/1 -> Delay8/1
